simulink model "StopWatch3_2018a"  (R2018a)
settings: Solver=VariableStepAuto  StartTime=0.0  StopTime=1.5  RelTol=1e-3
undefined symbols (not defined in the file or in its folder): sigbuilder_block
settings Model: Creator=86188  LastModifiedBy=bzhan

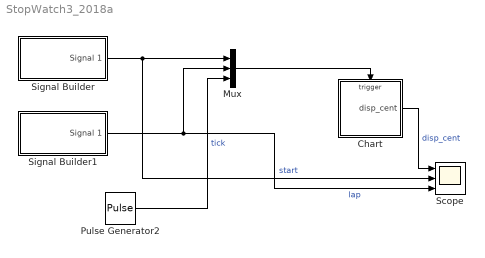
== system StopWatch3_2018a ==
  Chart : Stateflow chart  TreatAsAtomicUnit=on
  Mux : Mux  Inputs=3
  Pulse Generator2 : DiscretePulseGenerator  PulseType=Time based  Period=0.01  PulseWidth=50
  Scope : Scope  NumInputPorts=3
  Signal Builder : Subsystem  Tag=STV Subsys  LoadFcn=sigbuilder_block('load');  StartFcn=sigbuilder_block('start');  StopFcn=sigbuilder_block('stop');  ClipboardFcn=sigbuilder_block('clipboard');  mask(Sigbuilder block){tuvar=[0:10]}
      mask help: Simulink:masks:SigbuilderBlock_MD
      mask init:
      | if ~strcmp(get_param(bdroot(gcbh),'SimulationStatus'),'stopped') tuvar = sigbuilder_block('maskInit'); end
      settings: CopyFcn=sigbuilder_block('copy');  DeleteFcn=sigbuilder_block('delete');  ModelCloseFcn=sigbuilder_block('modelClose');  PreSaveFcn=sigbuilder_block('preSave');  PauseFcn=sigbuilder_block('pause');  ContinueFcn=sigbuilder_block('continue');  NameChangeFcn=sigbuilder_block('namechange');  OpenFcn=sigbuilder_block('open',[5.5 30 949 419 ]);  CloseFcn=sigbuilder_block('close');
      mask Display: plot(0, 0, 100, 100,[2, 2, 32, 32, 2], [68, 8, 8, 68, 68],[32, 2], [38, 38], [32, 19, 2],[53, 60, 44], [32, 17, 17, 2],[16, 16, 31, 31]);txt = getActiveGroup(gcbh);text(2, 100, txt,'verticalAlignment', 'top');
  Signal Builder1 : Subsystem  Tag=STV Subsys  LoadFcn=sigbuilder_block('load');  StartFcn=sigbuilder_block('start');  StopFcn=sigbuilder_block('stop');  ClipboardFcn=sigbuilder_block('clipboard');  mask(Sigbuilder block){tuvar=[0:10]}
      mask help: Simulink:masks:SigbuilderBlock_MD
      mask init:
      | if ~strcmp(get_param(bdroot(gcbh),'SimulationStatus'),'stopped') tuvar = sigbuilder_block('maskInit'); end
      settings: CopyFcn=sigbuilder_block('copy');  DeleteFcn=sigbuilder_block('delete');  ModelCloseFcn=sigbuilder_block('modelClose');  PreSaveFcn=sigbuilder_block('preSave');  PauseFcn=sigbuilder_block('pause');  ContinueFcn=sigbuilder_block('continue');  NameChangeFcn=sigbuilder_block('namechange');  OpenFcn=sigbuilder_block('open',[5.5 5.5 949 475 ]);  CloseFcn=sigbuilder_block('close');
      mask Display: plot(0, 0, 100, 100,[2, 2, 32, 32, 2], [68, 8, 8, 68, 68],[32, 2], [38, 38], [32, 19, 2],[53, 60, 44], [32, 17, 17, 2],[16, 16, 31, 31]);txt = getActiveGroup(gcbh);text(2, 100, txt,'verticalAlignment', 'top');
  wires:
  Signal Builder/1(Signal 1) -> Scope/2, Mux/1  "start"
  Signal Builder1/1(Signal 1) -> Scope/3, Mux/2  "lap"
  Mux/1 -> Chart/Trigger
  Pulse Generator2/1 -> Mux/3  "tick"
  Chart/1(disp_cent) -> Scope/1  "disp_cent"

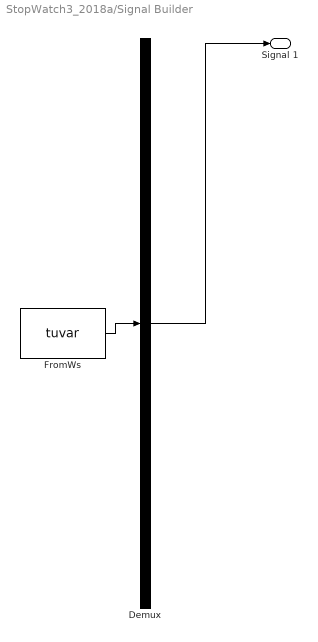
== system StopWatch3_2018a/Signal Builder ==
  Demux : Demux  Tag=STV Demux  Outputs=1
      settings: DisplayOption=none
  FromWs : FromWorkspace  Tag=STV FromWs  VariableName=tuvar
      SigBuilderData=|
      | common.afterFinalStr = 'Extrapolate'
      | common.sampleTime = 0
      | dataSet.timeRange = [0 10]
      | dataSet.name = 'Group 1'
      | sbobj.Groups.Name = 'Group 1'
      | sbobj.Groups.Signals.Name = 'Signal 1'
      | sbobj.Groups.Signals.XData = [0 0.05 0.05 0.3 0.3 0.4 0.4 0.6 0.6 0.7 0.7 0.9 0.9 10]
      | sbobj.Groups.Signals.YData = [0 0 1 1 0 0 1 1 0 0 1 1 0 0]
  Signal 1 : Outport  Tag=STV Outport  VectorParamsAs1DForOutWhenUnconnected=off
  wires:
  Demux/1 -> Signal 1/1
  FromWs/1 -> Demux/1

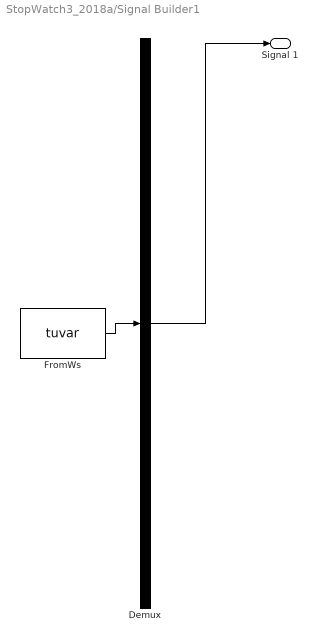
== system StopWatch3_2018a/Signal Builder1 ==
  Demux : Demux  Tag=STV Demux  Outputs=1
      settings: DisplayOption=none
  FromWs : FromWorkspace  Tag=STV FromWs  VariableName=tuvar
      SigBuilderData=|
      | common.afterFinalStr = 'Extrapolate'
      | common.sampleTime = 0
      | dataSet.timeRange = [0 10]
      | dataSet.name = 'Group 1'
      | sbobj.Groups.Name = 'Group 1'
      | sbobj.Groups.Signals.Name = 'Signal 1'
      | sbobj.Groups.Signals.XData = [0 0.1 0.1 0.2 0.2 0.3 0.3 0.4 0.4 10]
      | sbobj.Groups.Signals.YData = [0 0 1 1 0 0 1 1 0 0]
  Signal 1 : Outport  Tag=STV Outport  VectorParamsAs1DForOutWhenUnconnected=off
  wires:
  Demux/1 -> Signal 1/1
  FromWs/1 -> Demux/1

== stateflow chart StopWatch3_2018a/Chart ==
  settings: executeAtInitialization=1
  state StopW
    state Reset
      Reset -> (junction 5) [order 1] : LAP{cent=0;sec=0;
          | mins=0;disp_cent=0;
          | disp_sec=0;disp_min=0;}
    state LapStop
    (default) -> Reset
    LapStop -> Reset [order 2] : LAP
  state RunW
    state Running
      during:
      disp_cent=cent;
      disp_sec=sec;
      disp_min=mins;
    state Lap
    RunW -> (junction 19) : TIC{cent=cent+1;}
    (junction 19) -> (junction 25) [order 2]
    (junction 19) -> (junction 21) [order 1] : [cent==100]{cent=0;sec=sec+1;}
    (junction 21) -> (junction 25) [order 2]
    (junction 21) -> (junction 25) [order 1] : [sec==60]{sec=0;mins=mins+1;}
    Running -> Lap [order 2] : LAP
    Lap -> Running [order 2] : LAP
  (default) -> StopW
  Reset -> Running [order 1] : START
  Running -> Reset [order 1] : START
  LapStop -> Lap [order 1] : START
  Lap -> LapStop [order 1] : START
  data: cent local =0; mins local =0; disp_min local; sec local =0; disp_sec local =0; disp_cent output
  events: START input RISING_EDGE_EVENT; LAP input RISING_EDGE_EVENT; TIC input RISING_EDGE_EVENT
